simulink model "Fig231"  (R2014b)
settings: Solver=ode3  StartTime=0.0  StopTime=10  FixedStep=2e-5  RelTol=1e-5
libraries: commchan3 x1, commsink2 x1, commrandsrc2 x1
settings Model: Creator=Dennis Silage  LastModifiedBy=Silage
settings DataIOCC: SignalLoggingSaveFormat=ModelDataLogs
settings OptimizationCC: ExpressionDepthLimit=2147483647  InitFltsAndDblsToZero=on
settings DebuggingCC: UnderspecifiedInitializationDetection=Classic  MergeDetectMultiDrivingBlocksExec=none  SolverPrmCheckMsg=none  FcnCallInpInsideContextMsg=UseLocalSettings  StateNameClashWarn=warning
settings GRTTargetCC: CombineOutputUpdateFcns=off  GRTInterface=on

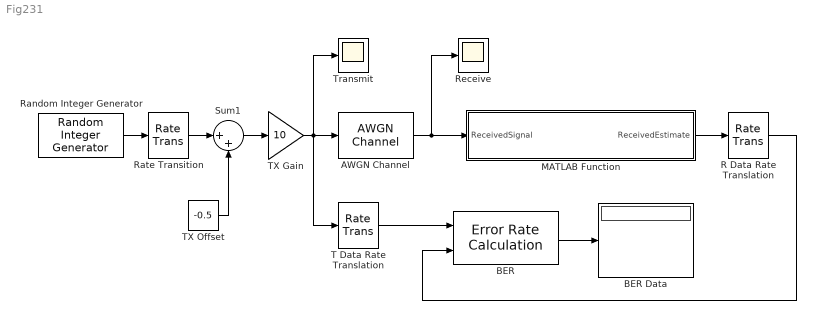
== system Fig231 ==
  AWGN Channel : commchan3/AWGN Channel  InputProcessing=Inherited (this choice will be removed - see release notes)  seed=randseed  noiseMode=Variance from mask  EbNodB=10  EsNodB=10  SNRdB=10  bitsPerSym=1  Ps=1  Tsym=1  variance=0
  BER : commsink2/Error Rate Calculation  N=1  st_delay=0  cp_mode=Entire frame  subframe=[]  PMode=Port  WsName=ErrorVec  RsMode2=off  stop=off  numErr=1  maxBits=1e6
  BER Data : Display
  MATLAB Function : MATLAB Function  TreatAsAtomicUnit=on
  R Data Rate Translation : RateTransition  OutPortSampleTime=1e-3
  Random Integer Generator : commrandsrc2/Random Integer Generator  mul=2  seed=37  Ts=1e-3  frameBased=off  sampPerFrame=50  orient=on  outDataType=double
  Rate Transition : RateTransition  OutPortSampleTime=2e-5
  Receive : Scope
      settings: TimeRange=0.05  YMin=-8  YMax=8  SaveName=ScopeData2
  Sum1 : Sum  Inputs=|++
  T Data Rate Translation : RateTransition  OutPortSampleTime=1e-3
  TX Gain : Gain  Gain=10
  TX Offset : Constant  Value=-0.5
  Transmit : Scope
      settings: TimeRange=0.05  YMin=-8  YMax=8
  wires:
  TX Gain/1 -> T Data Rate Translation/1, Transmit/1, AWGN Channel/1
  Random Integer Generator/1 -> Rate Transition/1
  Rate Transition/1 -> Sum1/1
  Sum1/1 -> TX Gain/1
  TX Offset/1 -> Sum1/2
  R Data Rate Translation/1 -> BER/2
  BER/1 -> BER Data/1
  T Data Rate Translation/1 -> BER/1
  AWGN Channel/1 -> MATLAB Function/1(ReceivedSignal), Receive/1
  MATLAB Function/1(ReceivedEstimate) -> R Data Rate Translation/1

== matlab function Fig231/MATLAB Function ==
  data: ReceivedSignal input; ReceivedEstimate output
function ReceivedEstimate = Multisampling(ReceivedSignal)
%#codegen
persistent RcvdEst flag PriorRcvdEst

if isempty(flag)
    flag = 0;
    RcvdEst = 0;
    PriorRcvdEst = 0;
end

flag = flag + 1;
ReceivedEstimate = PriorRcvdEst;

if (flag == 50)
    flag = 0;
    ReceivedEstimate = 5 * sign(RcvdEst);
    RcvdEst = 0;
    PriorRcvdEst = ReceivedEstimate;
elseif (mod(flag, 3) == 0 && flag ~= 48) 
    RcvdEst = RcvdEst + sign(ReceivedSignal);
end
end
